simulink model "sl_ctorqueTraj_og"  (R2014a)
settings: Solver=ode45  StartTime=0.0  StopTime=10  FixedStep=0.01  MaxStep=0.05  RelTol=1e-3
PreLoadFcn:
  | puma560
  | p560 = nofriction(p560);
libraries: roblocks x3
settings Model: ExtModeTrigMode=oneshot  ExtModeArmWhenConnect=off  Creator=pic  LastModifiedBy=MRDLAB
settings SolverCC: ZeroCrossControl=DisableAll
settings DataIOCC: LimitDataPoints=off  SignalLoggingSaveFormat=ModelDataLogs  ReturnWorkspaceOutputs=on
settings OptimizationCC: BlockReduction=off  BooleanDataType=off  ExpressionDepthLimit=2147483647  InitFltsAndDblsToZero=on
settings DebuggingCC: SaveWithParameterizedLinksMsg=none  UnderspecifiedInitializationDetection=Classic  SignalResolutionControl=TryResolveAllWithWarning  SolverPrmCheckMsg=none  MultiTaskDSMMsg=warning  MultiTaskCondExecSysMsg=none  FcnCallInpInsideContextMsg=UseLocalSettings  StateNameClashWarn=warning
settings HardwareCC: TargetUnknown=on
settings RTWCC: IncludeERTFirstTime=on
settings GRTTargetCC: ModelReferenceCompliant=off  CompOptLevelCompliant=off  CombineOutputUpdateFcns=off  MatFileLogging=off  GRTInterface=on

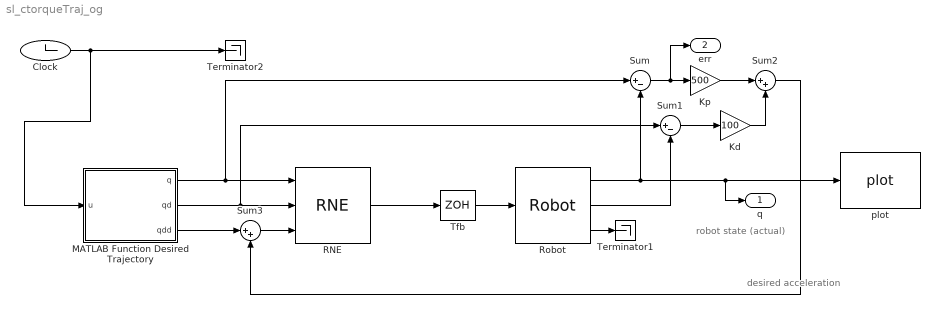
== system sl_ctorqueTraj_og ==
  note: robot state
      | (actual)
  note: desired acceleration
  Clock : Clock
  Kd : Gain  Gain=100  SaturateOnIntegerOverflow=on  OutDataTypeStr=Inherit: Same as input  ParamDataTypeStr=Inherit: Same as input
  Kp : Gain  Gain=500  SaturateOnIntegerOverflow=on  OutDataTypeStr=Inherit: Same as input  ParamDataTypeStr=Inherit: Same as input
  MATLAB Function Desired Trajectory : MATLAB Function  TreatAsAtomicUnit=on
  RNE : roblocks/Dynamics/RNE  robot=myRobot  grav=[0 0 9.81]
  Robot : roblocks/Dynamics/Robot  robot=myRobot  q0=[0 0 0 0 0 0]
  Sum : Sum  Inputs=|+-  SaturateOnIntegerOverflow=on  InputSameDT=on  OutDataTypeStr=Inherit: Same as first input
  Sum1 : Sum  Inputs=|+-  SaturateOnIntegerOverflow=on  InputSameDT=on  OutDataTypeStr=Inherit: Same as first input
  Sum2 : Sum  Inputs=|++  SaturateOnIntegerOverflow=on  InputSameDT=on  OutDataTypeStr=Inherit: Same as first input
  Sum3 : Sum  Inputs=|++  SaturateOnIntegerOverflow=on  InputSameDT=on  OutDataTypeStr=Inherit: Same as first input
  Terminator1 : Terminator
  Terminator2 : Terminator
  Tfb : ZeroOrderHold  SampleTime=0.01
  plot : roblocks/Robot Graphics/plot  robot=myRobot  fps=25  holdplot=on
  q : Outport
  err : Outport  Port=2
  wires:
  Sum/1 -> Kp/1, err/1
  Kp/1 -> Sum2/1
  Robot/1 -> Sum/2, q/1, plot/1
  Robot/2 -> Sum1/2
  RNE/1 -> Tfb/1
  MATLAB Function Desired Trajectory/1(q) -> Sum/1, RNE/1
  MATLAB Function Desired Trajectory/2(qd) -> Sum1/1, RNE/2
  Sum1/1 -> Kd/1
  Kd/1 -> Sum2/2
  MATLAB Function Desired Trajectory/3(qdd) -> Sum3/1
  Robot/3 -> Terminator1/1
  Clock/1 -> MATLAB Function Desired Trajectory/1(u), Terminator2/1
  Sum3/1 -> RNE/3
  Sum2/1 -> Sum3/2
  Tfb/1 -> Robot/1

== matlab function sl_ctorqueTraj_og/MATLAB Function Desired Trajectory ==
  data: u input; q output; qd output; qdd output
% writen by Tim K. for ME 8287. 2015
% Allows creation of a trajectory as a function of time.  All code 
% should be self containted.
% input - time in sec
% output - joint angle, velocity, and acceleration : q, qd, qdd
function [q,qd,qdd ] = desiredTrajectory(u)
%#codegen

t = u(1);  % sample time
A = 0.05;  % amplitude/circle radius
k = 1;  % speed
z = 0.5;

%               x                y        z | orientation
q   = [      A*sin(k*t)       A*cos(k*t)  z     0 0 0   ]'; 
qd  = [    k*A*cos(k*t)    -k*A*sin(k*t)  0     0 0 0   ]'; 
qdd = [ -k^2*A*sin(k*t)  -k^2*A*cos(k*t)  0     0 0 0   ]';
